simulink model "Cascade_Realization"  (R2020b)
settings: Solver=VariableStepAuto  StartTime=0.0  StopTime=10.0  RelTol=1e-3
settings Model: Creator=vijay jagtap  LastModifiedBy=vijay jagtap

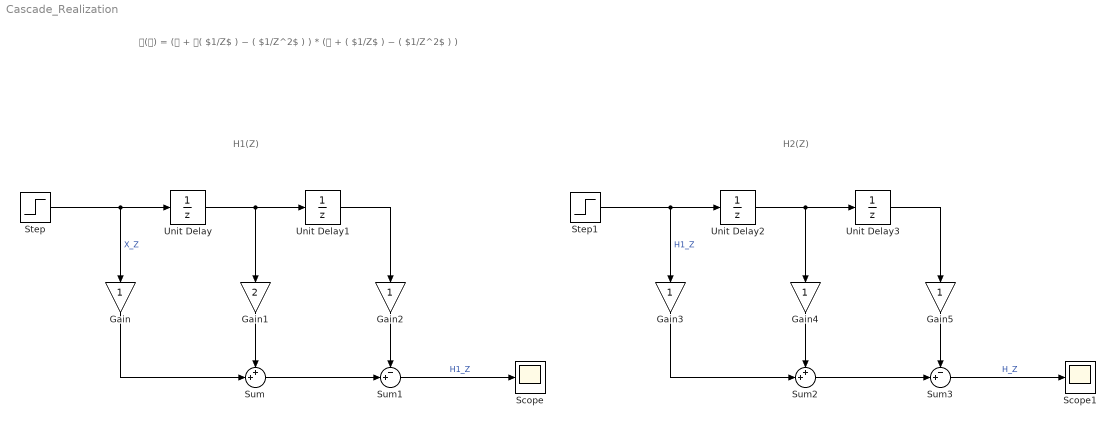
== system Cascade_Realization ==
  note: H2(Z)
  note: 𝐇(𝐳) = (𝟏 + 𝟐( $1/Z$ ) − ( $1/Z^2$ ) ) * (𝟏 + ( $1/Z$ ) − ( $1/Z^2$ ) )
  note: H1(Z)
  Gain{,2..5} (5 alike) : Gain
  Gain1 : Gain  Gain=2
  Scope : Scope
  Scope1 : Scope
  Step : Step  SampleTime=0
  Step1 : Step  SampleTime=0
  Sum : Sum  Inputs=++|
  Sum1 : Sum  Inputs=-+|
  Sum2 : Sum  Inputs=++|
  Sum3 : Sum  Inputs=-+|
  Unit Delay{,1..3} (4 alike) : UnitDelay  SampleTime=-1  HasFrameUpgradeWarning=on
  wires:
  Step/1 -> Gain/1, Unit Delay/1  "X_Z"
  Unit Delay/1 -> Gain1/1, Unit Delay1/1
  Unit Delay1/1 -> Gain2/1
  Gain1/1 -> Sum/1
  Gain/1 -> Sum/2
  Sum/1 -> Sum1/2
  Gain2/1 -> Sum1/1
  Sum1/1 -> Scope/1  "H1_Z"
  Unit Delay2/1 -> Gain4/1, Unit Delay3/1
  Sum3/1 -> Scope1/1  "H_Z"
  Unit Delay3/1 -> Gain5/1
  Gain4/1 -> Sum2/1
  Gain5/1 -> Sum3/1
  Sum2/1 -> Sum3/2
  Gain3/1 -> Sum2/2
  Step1/1 -> Gain3/1, Unit Delay2/1  "H1_Z"
